simulink model "TTS3_Controller"  (R2019b)
settings: Solver=VariableStepAuto  StartTime=0.0  StopTime=10.0  FixedStep=Ts  RelTol=1e-3
PostLoadFcn:
  | if any(exist('dsrtsu_mdlpostloadfcn', 'file') ~= 0), dsrtsu_mdlpostloadfcn('Execute', bdroot); end
undefined symbols (not defined in the file): Valve_LD_posref, Valve_MD_posref, Valve_RD_posref
libraries: simulink x1
settings Model: DSRTSU_INTERNAL_RTI_VER=550  DSRTSU_INTERNAL_RTI_TYPE=rti1104  RTICANMMDATA=struct('GeneralSetupData',struct('modelroot','E:\Will\integration-project-5sc26\Teacher_files','generalsettings',struct('filesettings',struct('destfolder',struct('Name','RTICANMM_FILES','Check',1),'buildfolder',struct('Name','.','Check',1),'AbsDestfolder',struct('Name','E:\Will\integration-project-5sc26\Teacher_files\RTICANMM_FILES'),'AbsBuildfolder',struct('Name','E:\Will\integration-project-5sc26\Teacher_files'))),'options',struct('addpaths',1,'rmpaths',1,'addtrcexclusion',true,'cannavigator',struct('checkmonitoring',0),'show_usrtrc',0,'use_usrtrc',0),'advanced',struct('options',ones(1,100)),'MPSetup',{{}},'RTI',struct('Type','RTI1104','Ver','7.13','Date','02-Nov-2019'),'modelname','RL_TTS3_Controller_Blank','block','RL_TTS3_Controller_Blank'))  DSRTSU_INTERNAL_RTIFPGA=150  Creator=whendrix  LastModifiedBy=alexg
settings OptimizationCC: BlockReduction=off  OptimizeBlockIOStorage=off  BufferReuse=off  GlobalBufferReuse=off  ExpressionFolding=off  LocalBlockOutputs=off  OptimizeDataStoreBuffers=off  BusAssignmentInplaceUpdate=off
settings DebuggingCC: BusObjectLabelMismatch=none
settings HardwareCC: ProdBitPerPointer=32  ProdBitPerSizeT=32  ProdBitPerPtrDiffT=32  ProdLargestAtomicInteger=Integer  ProdEndianess=BigEndian  ProdWordSize=32  ProdHWDeviceType=Custom Processor->Custom  TargetIntDivRoundTo=Zero  TargetEndianess=BigEndian  TargetHWDeviceType=Custom Processor->Custom
settings ModelReferenceCC: ModelReferenceNumInstancesAllowed=Single  ModelReferenceMinAlgLoopOccurrences=on
settings SFSimCC: MATLABDynamicMemAlloc=off  CustomCodeUndefinedFunction=UseInterfaceOnly
settings RTWCC: Description=dSPACE DS1104 Hardware Platform  SystemTargetFile=rti1104.tlc  MakeCommand=make_rti  TemplateMakefile=rti1104.tmf
settings CodeAppCC: MaxIdLength=63
settings STFCustomTargetCC: ParMdlRefBuildCompliant=on  SystemTargetFile=rti1104.tlc
settings GRTTargetCC: TargetLangStandard=C89/C90 (ANSI)  CompOptLevelCompliant=off  ConcurrentExecutionCompliant=off  CombineOutputUpdateFcns=off  MatFileLogging=off  CPPClassGenCompliant=off  UseToolchainInfoCompliant=off

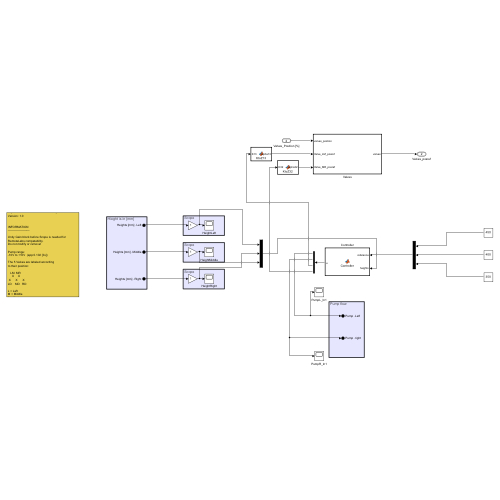
[thumbnail: Simulink's stored preview of the top-level diagram]
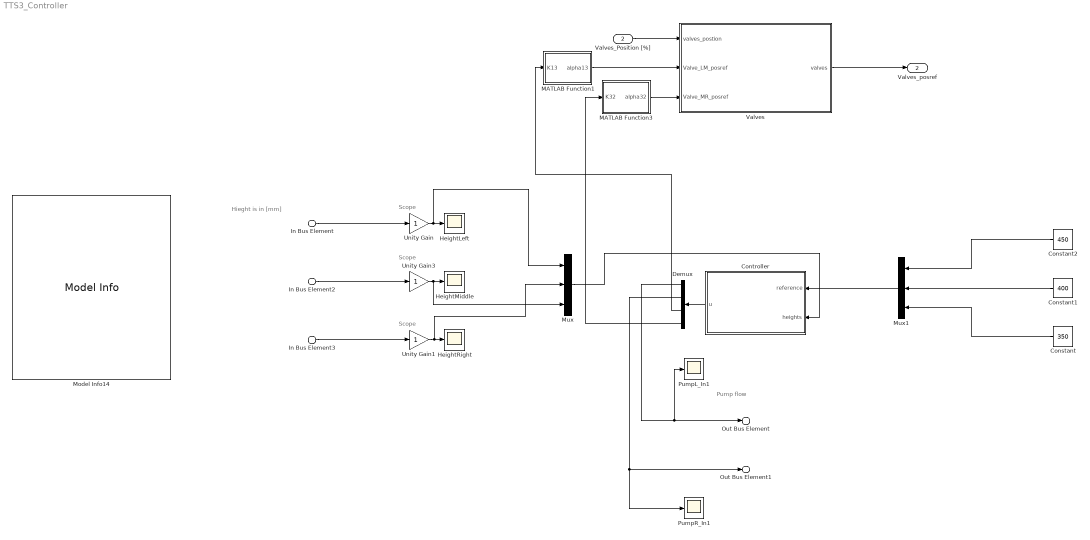
== system TTS3_Controller ==
  note: Pump flow
  note: Hieght is in [mm]
  note: Scope
  note: Scope
  note: Scope
  In Bus Element3 : Inport  PortName=Heights [mm]  Element=Right
  In Bus Element2 : Inport  PortName=Heights [mm]  Element=Middle
  In Bus Element : Inport  PortName=Heights [mm]  Element=Left
  Valves_Position [%] : Inport  Port=2  OutDataTypeStr=Bus: ValvesSOCI
  Constant : Constant  Value=350  SampleTime=0.1
  Constant1 : Constant  Value=400  SampleTime=0.1
  Constant2 : Constant  Value=450  SampleTime=0.1
  Controller : MATLAB Function  TreatAsAtomicUnit=on
  Demux : Demux
  HeightLeft : Scope
  HeightMiddle : Scope
  HeightRight : Scope
  MATLAB Function1 : MATLAB Function  TreatAsAtomicUnit=on
  MATLAB Function3 : MATLAB Function  TreatAsAtomicUnit=on
  Model Info14 : simulink/Model-Wide Utilities/Model Info  Frame=on  DisplayStringWithTags=|  HorizontalTextAlignment=Left  LeftAlignmentValue=0.02
      | Start model for the "Three Tank"
      | experiment on the "Three Tank" setup.
      | Version: 1.0
      | 
      | 
      | INFORMATION
      | ----------------------
      | 
      | Unity Gain block before Scope is needed for
      | RemoteLabs compatebility. 
      | Do not modify or remove!
      | 
      | Pump range:
      | -10V to +10V  (app 0.102 [l/s])
      | 
      | The 5 Valves are labeled according 
      | to their position:
      | 
      |    LM  MR
      |      X     X
      |  X      X      X
      | LD    MD   RD
      | 
      | L = Left
      | M = Middle
      | R = Right
      | D = Down
  Mux : Mux  Inputs=3
  Mux1 : Mux  Inputs=3
  PumpL_In1 : Scope
  PumpR_In1 : Scope
  Unity Gain : Gain
  Unity Gain1 : Gain
  Unity Gain3 : Gain
  Valves : Subsystem  TreatAsAtomicUnit=on
  Out Bus Element1 : Outport  VectorParamsAs1DForOutWhenUnconnected=off  PortName=Pump  Element=right
  Out Bus Element : Outport  VectorParamsAs1DForOutWhenUnconnected=off  PortName=Pump  Element=Left
  Valves_posref : Outport  Port=2  OutDataTypeStr=Bus: ValveSICO
  wires:
  Unity Gain/1 -> Mux/1, HeightLeft/1
  Unity Gain3/1 -> HeightMiddle/1, Mux/3
  Unity Gain1/1 -> Mux/2, HeightRight/1
  Demux/1 -> Out Bus Element/1, PumpL_In1/1
  In Bus Element/1 -> Unity Gain/1
  In Bus Element2/1 -> Unity Gain3/1
  In Bus Element3/1 -> Unity Gain1/1
  Valves_Position [%]/1 -> Valves/1(valves_postion)
  Valves/1(valves) -> Valves_posref/1
  Mux/1 -> Controller/2(heights)
  Demux/3 -> MATLAB Function1/1(K13)
  Demux/4 -> MATLAB Function3/1(K32)
  Controller/1(u) -> Demux/1
  Constant/1 -> Mux1/3
  Mux1/1 -> Controller/1(reference)
  Constant2/1 -> Mux1/1
  Constant1/1 -> Mux1/2
  MATLAB Function1/1(alpha13) -> Valves/2(Valve_LM_posref)
  MATLAB Function3/1(alpha32) -> Valves/3(Valve_MR_posref)
  Demux/2 -> Out Bus Element1/1, PumpR_In1/1

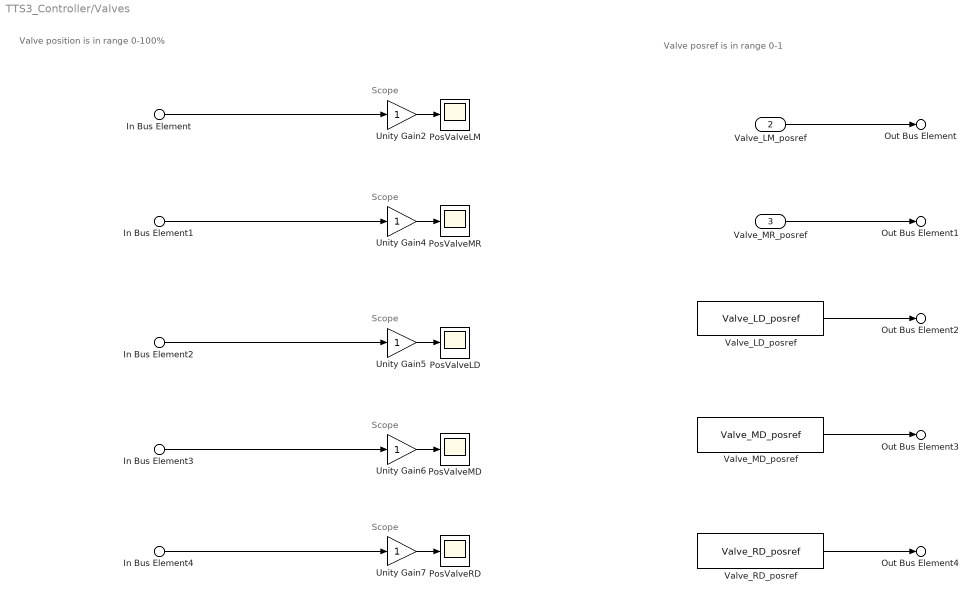
== system TTS3_Controller/Valves ==
  note: Valve posref is in range 0-1
  note: Valve position is in range 0-100%
  note: Scope
  note: Scope
  note: Scope
  note: Scope
  note: Scope
  In Bus Element : Inport  PortName=valves_postion  Element=LM_pos
  In Bus Element1 : Inport  PortName=valves_postion  Element=MR_pos
  In Bus Element4 : Inport  PortName=valves_postion  Element=RD_pos
  In Bus Element3 : Inport  PortName=valves_postion  Element=MD_pos
  In Bus Element2 : Inport  PortName=valves_postion  Element=LD_pos
  Valve_LM_posref : Inport  Port=2
  Valve_MR_posref : Inport  Port=3
  PosValveLD : Scope
  PosValveLM : Scope
  PosValveMD : Scope
  PosValveMR : Scope
  PosValveRD : Scope
  Unity Gain{2,4..7} (5 alike) : Gain
  Valve_LD_posref : Constant  Value=Valve_LD_posref
  Valve_MD_posref : Constant  Value=Valve_MD_posref
  Valve_RD_posref : Constant  Value=Valve_RD_posref
  Out Bus Element : Outport  PortName=valves  Element=LM_posref
  Out Bus Element1 : Outport  PortName=valves  Element=MR_posref
  Out Bus Element3 : Outport  PortName=valves  Element=MD_posref
  Out Bus Element4 : Outport  PortName=valves  Element=RD_posref
  Out Bus Element2 : Outport  PortName=valves  Element=LD_posref
  wires:
  Unity Gain6/1 -> PosValveMD/1
  Unity Gain7/1 -> PosValveRD/1
  Unity Gain4/1 -> PosValveMR/1
  Unity Gain5/1 -> PosValveLD/1
  Unity Gain2/1 -> PosValveLM/1
  In Bus Element/1 -> Unity Gain2/1
  In Bus Element1/1 -> Unity Gain4/1
  In Bus Element2/1 -> Unity Gain5/1
  In Bus Element3/1 -> Unity Gain6/1
  In Bus Element4/1 -> Unity Gain7/1
  Valve_LM_posref/1 -> Out Bus Element/1
  Valve_MD_posref/1 -> Out Bus Element3/1
  Valve_RD_posref/1 -> Out Bus Element4/1
  Valve_MR_posref/1 -> Out Bus Element1/1
  Valve_LD_posref/1 -> Out Bus Element2/1

== matlab function TTS3_Controller/MATLAB Function1 ==
  data: K13 input; alpha13 output
function alpha13 = KtoZ13(K13)
% [0,0.24] -> [-50,50]
    a13 = 2.409;
    b13 = 9.583;
    c13 = 4.241;
    d13 = 9.07;
    e13 = -0.01094;
    temp = (a13/(K13-e13) -b13)/c13;
    if temp < 0
        temp = 1e-4;
    end

    alpha13 = log(temp)/-d13 + 0.5; %[0 ~ 1]
%     alpha13 = alpha13*100;

end

== matlab function TTS3_Controller/Controller ==
  data: reference input; heights input; u output
function u = Controller(reference, heights)

% reference = [450, 400, 359]
% height = [h1, h2, h3]
% u = [p1, p2, k13, k32]

K = [1.26583363863119	0.0603891831825281	0.700331838202608;
0.0652453998465126	1.21560150893254	0.363852113183011;
-0.0863846849137246	0.0424057591826027	0.494138459597246;
0.0694700898243913	-0.0849004586324254	0.388724208913166];

reference = [reference(1); reference(2); reference(3)];
heights = [heights(1); heights(2); heights(3)];

% Error calculation
error = reference - heights;

% Control input calculation
u = K * error;

end

== matlab function TTS3_Controller/MATLAB Function3 ==
  data: K32 input; alpha32 output
function alpha32 = KtoZ32(K32)
    a32 = -2.145;
    b32 = -8.547;
    c32 = -3.072;
    d32 = 8.984;
    e32 = -0.01151;
    temp = (a32/(K32-e32) -b32)/c32;
    if temp < 0
        temp = 1e-4;
    end
    alpha32 = log(temp)/-d32 + 0.5;%[0 ~ 1]
%     alpha32 = alpha32*100;
end
